simulink model "grid_2021a"  (R2021a)
settings: Solver=VariableStepAuto  StartTime=0.1  StopTime=40  RelTol=1e-3
values from neighbouring files (symbols this model uses):
  close_time = 40    [params.m]
  J_eol = 2*H_tot*P_nom/w_eol_nom^2    (= 921600)    [wind_params.m]
  M1 = M1_backup    [automation.m]    (also in params.m = Machine)
  M2 = M1    [automation.m]    (also in params.m = Machine)
  omega_tab = v_vent_tab*lambda_opt/R_pal    [wind_params.m]
  open_time = 80    [params.m]
  P_eol = P_ren - P_sol    [automation.m]
  P_sol = Power_per_pannel * round((0.6 * P_ren)/ Power_per_pannel)    [automation.m]    (also in params_solar.m = 1000000)
  Pn_L1 = M1.P0 + M2.P0 + P_ren    [automation.m]    (also in params.m = M1.P0 + M2.P0)
  Pn_L2 = Pn_L1 * 0.01    [automation.m]    (also in params.m = Pn_L1 * 0.2)
  Power_per_pannel = 383    [params_battery.m]    (also in params_solar.m = 180.43249709)
  R_pal = 24    [wind_params.m]
  ref_volt = 4160    [params.m]
  ro_air = 1.22    [wind_params.m]
  S_pal = pi*R_pal*R_pal    (= 1809.55736847)    [wind_params.m]
  Ts = 2e-4    (= 0.0002)    [params_solar.m]
  w_eol_nom = v_pal_nom/R_pal    (= 3.125)    [wind_params.m]
  w_zero = 3.000    (= 3)    [wind_params.m]
undefined symbols (not defined in the file or in its folder): Cp_ref, P_eol_base, P_opt_tab2
libraries: nesl_utility x45, fl_lib x43, ee_lib x27
(part 2 of 2)

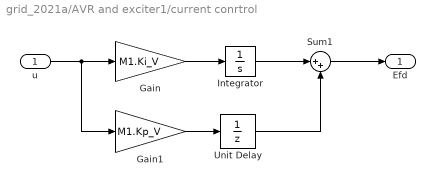
== system grid_2021a/AVR and exciter1/current conrtrol ==
  u : Inport
  Gain : Gain  Gain=M1.Ki_V
  Gain1 : Gain  Gain=M1.Kp_V
  Integrator : Integrator
  Sum1 : Sum  Inputs=|++
  Unit Delay : UnitDelay  InitialCondition=1  SampleTime=-1  HasFrameUpgradeWarning=on
  Efd : Outport
  wires:
  u/1 -> Gain1/1, Gain/1
  Sum1/1 -> Efd/1
  Gain/1 -> Integrator/1
  Integrator/1 -> Sum1/1
  Gain1/1 -> Unit Delay/1
  Unit Delay/1 -> Sum1/2

== system grid_2021a/AVR and exciter2/current conrtrol ==
  u : Inport
  Gain : Gain  Gain=M2.Ki_V
  Gain1 : Gain  Gain=M2.Kp_V
  Integrator : Integrator
  Sum1 : Sum  Inputs=|++
  Unit Delay : UnitDelay  InitialCondition=1  SampleTime=-1  HasFrameUpgradeWarning=on
  Efd : Outport
  wires:
  u/1 -> Gain1/1, Gain/1
  Sum1/1 -> Efd/1
  Gain/1 -> Integrator/1
  Integrator/1 -> Sum1/1
  Gain1/1 -> Unit Delay/1
  Unit Delay/1 -> Sum1/2

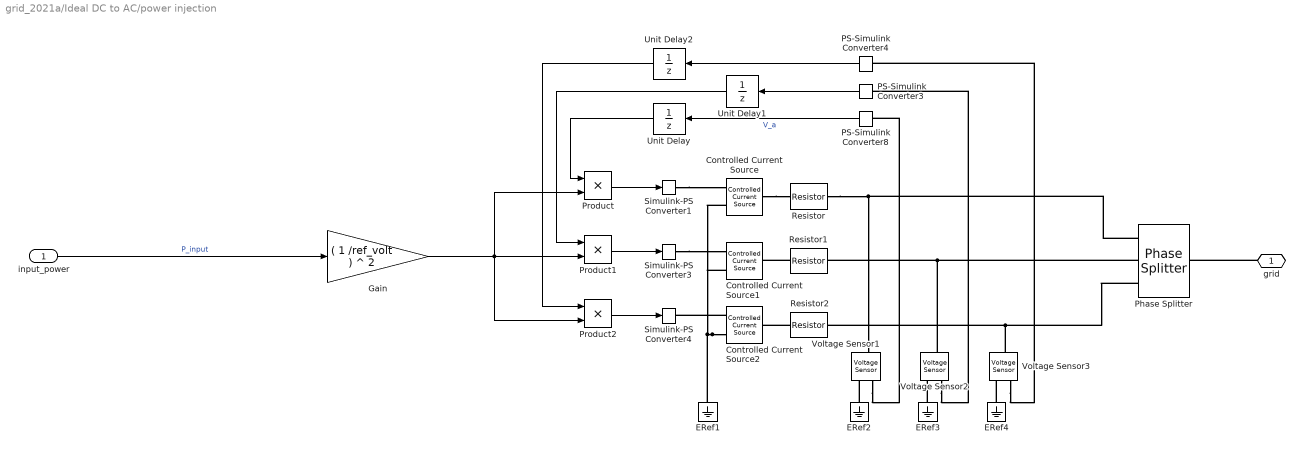
== system grid_2021a/Ideal DC to AC/power injection ==
  input_power : Inport
  Controlled Current Source : fl_lib/Electrical/Electrical Sources/Controlled Current Source
  Controlled Current Source1 : fl_lib/Electrical/Electrical Sources/Controlled Current Source
  Controlled Current Source2 : fl_lib/Electrical/Electrical Sources/Controlled Current Source
  ERef{1..4} (4 alike) : fl_lib/Electrical/Electrical Elements/Electrical Reference
  Gain : Gain  Gain=( 1 /ref_volt ) ^ 2
  PS-Simulink Converter3 : nesl_utility/PS-Simulink Converter  PhysicalDomain=network_engine_domain  SubClassName=ps_output  LeftPortType=input  RightPortType=output  PseudoPeriodic=off  Frequencies=[]  VectorFormat=1-D array  Unit=inherit  AffineConversion=off
  PS-Simulink Converter4 : nesl_utility/PS-Simulink Converter  PhysicalDomain=network_engine_domain  SubClassName=ps_output  LeftPortType=input  RightPortType=output  PseudoPeriodic=off  Frequencies=[]  VectorFormat=1-D array  Unit=inherit  AffineConversion=off
  PS-Simulink Converter8 : nesl_utility/PS-Simulink Converter  PhysicalDomain=network_engine_domain  SubClassName=ps_output  LeftPortType=input  RightPortType=output  PseudoPeriodic=off  Frequencies=[]  VectorFormat=1-D array  Unit=inherit  AffineConversion=off
  Phase Splitter : ee_lib/Connectors & References/Phase Splitter
  Product : Product
  Product1 : Product
  Product2 : Product
  Resistor : fl_lib/Electrical/Electrical Elements/Resistor  R=1e-6 Ohm  i_specify=off  i_priority=None  i=0 A  i_nominal_specify=off  i_nominal_unit=A  i_nominal_value=1  v_specify=off  v_priority=None  v=0 V  v_nominal_specify=off  v_nominal_unit=V  v_nominal_value=1
  Resistor1 : fl_lib/Electrical/Electrical Elements/Resistor  R=1e-6 Ohm  i_specify=off  i_priority=None  i=0 A  i_nominal_specify=off  i_nominal_unit=A  i_nominal_value=1  v_specify=off  v_priority=None  v=0 V  v_nominal_specify=off  v_nominal_unit=V  v_nominal_value=1
  Resistor2 : fl_lib/Electrical/Electrical Elements/Resistor  R=1e-6 Ohm  i_specify=off  i_priority=None  i=0 A  i_nominal_specify=off  i_nominal_unit=A  i_nominal_value=1  v_specify=off  v_priority=None  v=0 V  v_nominal_specify=off  v_nominal_unit=V  v_nominal_value=1
  Simulink-PS Converter1 : nesl_utility/Simulink-PS Converter  PhysicalDomain=network_engine_domain  SubClassName=ps_input  LeftPortType=input  RightPortType=output  PseudoPeriodic=off  Frequencies=[]  NoiseDistribution=none  NoiseParameters=[]  Unit=1  AffineConversion=off  FilteringAndDerivatives=filter  SimscapeFilterOrder=1  InputFilterTimeConstant=0.0001  UdotUserProvided=0
  Simulink-PS Converter3 : nesl_utility/Simulink-PS Converter  PhysicalDomain=network_engine_domain  SubClassName=ps_input  LeftPortType=input  RightPortType=output  PseudoPeriodic=off  Frequencies=[]  NoiseDistribution=none  NoiseParameters=[]  Unit=1  AffineConversion=off  FilteringAndDerivatives=filter  SimscapeFilterOrder=1  InputFilterTimeConstant=0.0001  UdotUserProvided=0
  Simulink-PS Converter4 : nesl_utility/Simulink-PS Converter  PhysicalDomain=network_engine_domain  SubClassName=ps_input  LeftPortType=input  RightPortType=output  PseudoPeriodic=off  Frequencies=[]  NoiseDistribution=none  NoiseParameters=[]  Unit=1  AffineConversion=off  FilteringAndDerivatives=filter  SimscapeFilterOrder=1  InputFilterTimeConstant=0.0001  UdotUserProvided=0
  Unit Delay : UnitDelay  SampleTime=-1  HasFrameUpgradeWarning=on
  Unit Delay1 : UnitDelay  SampleTime=-1  HasFrameUpgradeWarning=on
  Unit Delay2 : UnitDelay  SampleTime=-1  HasFrameUpgradeWarning=on
  Voltage Sensor1 : fl_lib/Electrical/Electrical Sensors/Voltage Sensor
  Voltage Sensor2 : fl_lib/Electrical/Electrical Sensors/Voltage Sensor
  Voltage Sensor3 : fl_lib/Electrical/Electrical Sensors/Voltage Sensor
  grid : PMIOPort  Side=Right
  wires:
  PS-Simulink Converter4/1 -> Unit Delay2/1
  PS-Simulink Converter8/1 -> Unit Delay/1  "V_a"
  PS-Simulink Converter3/1 -> Unit Delay1/1
  Product/1 -> Simulink-PS Converter1/1
  Product1/1 -> Simulink-PS Converter3/1
  Product2/1 -> Simulink-PS Converter4/1
  Unit Delay/1 -> Product/1
  Unit Delay1/1 -> Product1/1
  Unit Delay2/1 -> Product2/1
  Gain/1 -> Product1/2, Product2/2, Product/2
  input_power/1 -> Gain/1  "P_input"
  connections:
  Resistor1/LConn1 -- Controlled Current Source1/LConn1
  Resistor2/LConn1 -- Controlled Current Source2/LConn1
  ERef2/LConn1 -- Voltage Sensor1/RConn2
  Controlled Current Source2/RConn2 -- ERef1/LConn1 -- Controlled Current Source/RConn2 -- Controlled Current Source1/RConn2
  Phase Splitter/RConn1 -- Resistor/RConn1 -- Voltage Sensor1/LConn1
  Simulink-PS Converter1/RConn1 -- Controlled Current Source/RConn1
  ERef4/LConn1 -- Voltage Sensor3/RConn2
  Controlled Current Source/LConn1 -- Resistor/LConn1
  Phase Splitter/RConn2 -- Resistor1/RConn1 -- Voltage Sensor2/LConn1
  Controlled Current Source2/RConn1 -- Simulink-PS Converter4/RConn1
  grid/RConn1 -- Phase Splitter/LConn1
  ERef3/LConn1 -- Voltage Sensor2/RConn2
  Phase Splitter/RConn3 -- Resistor2/RConn1 -- Voltage Sensor3/LConn1
  Simulink-PS Converter3/RConn1 -- Controlled Current Source1/RConn1
  Voltage Sensor1/RConn1 -- PS-Simulink Converter8/LConn1
  Voltage Sensor2/RConn1 -- PS-Simulink Converter3/LConn1
  Voltage Sensor3/RConn1 -- PS-Simulink Converter4/LConn1

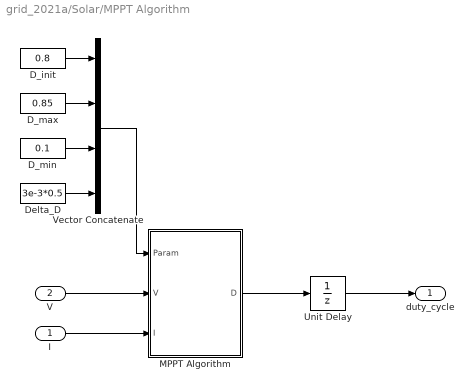
== system grid_2021a/Solar/MPPT Algorithm ==
  I : Inport
  V : Inport  Port=2
  D_init : Constant  Value=0.8
  D_max : Constant  Value=0.85
  D_min : Constant  Value=0.1
  Delta_D : Constant  Value=3e-3*0.5
  MPPT Algorithm : MATLAB Function  SystemSampleTime=Ts
  Unit Delay : UnitDelay  InitialCondition=0.85  SampleTime=-1  HasFrameUpgradeWarning=on
  Vector Concatenate : Concatenate  NumInputs=4
  duty_cycle : Outport
  wires:
  V/1 -> MPPT Algorithm/2(V)
  Vector Concatenate/1 -> MPPT Algorithm/1(Param)
  D_max/1 -> Vector Concatenate/2
  D_init/1 -> Vector Concatenate/1
  D_min/1 -> Vector Concatenate/3
  MPPT Algorithm/1(D) -> Unit Delay/1
  Delta_D/1 -> Vector Concatenate/4
  I/1 -> MPPT Algorithm/3(I)
  Unit Delay/1 -> duty_cycle/1

== system grid_2021a/Solar/Sensing Current ==
  Current Sensor : fl_lib/Electrical/Electrical Sensors/Current Sensor
  PS-Simulink/I : nesl_utility/PS-Simulink Converter  PhysicalDomain=network_engine_domain  SubClassName=ps_output  LeftPortType=input  RightPortType=output  PseudoPeriodic=off  Frequencies=[]  VectorFormat=1-D array  Unit=1  AffineConversion=off
  + : PMIOPort  Side=Left
  - : PMIOPort  Port=2  Side=Right
  I : Outport
  wires:
  PS-Simulink/I/1 -> I/1
  connections:
  -/RConn1 -- Current Sensor/RConn2
  Current Sensor/LConn1 -- +/RConn1
  Current Sensor/RConn1 -- PS-Simulink/I/LConn1

== system grid_2021a/Solar/sensing voltage ==
  PS-Simulink Converter : nesl_utility/PS-Simulink Converter  PhysicalDomain=network_engine_domain  SubClassName=ps_output  LeftPortType=input  RightPortType=output  PseudoPeriodic=off  Frequencies=[]  VectorFormat=1-D array  Unit=inherit  AffineConversion=off
  Voltage Sensor : fl_lib/Electrical/Electrical Sensors/Voltage Sensor
  + : PMIOPort  Side=Left
  - : PMIOPort  Port=2  Side=Right
  V : Outport
  wires:
  PS-Simulink Converter/1 -> V/1
  connections:
  Voltage Sensor/LConn1 -- +/RConn1
  Voltage Sensor/RConn2 -- -/RConn1
  Voltage Sensor/RConn1 -- PS-Simulink Converter/LConn1

== system grid_2021a/Wind turbine/Pitch control ==
  In1 : Inport
  In2 : Inport  Port=2
  Gain1 : Gain  Gain=-200
  Saturation : Saturate  UpperLimit=inf  LowerLimit=0
  Sum1 : Sum  Inputs=|+-
  Out1 : Outport
  wires:
  In2/1 -> Sum1/2
  Gain1/1 -> Saturation/1
  Sum1/1 -> Gain1/1
  In1/1 -> Sum1/1
  Saturation/1 -> Out1/1

== matlab function grid_2021a/Solar/MPPT Algorithm/MPPT Algorithm ==
  settings: updateMethod=DISCRETE  sampleTime=Ts_DC
  data: Param input; V input; I input; D output
function D  = PandO(Param, V, I)

% MPPT controller based on the Perturb & Observe algorithm.

% D output = Duty cycle of the boost converter (value between 0 and 1)
%
% V input = PV array terminal voltage (V)
% I input = PV array current (A)
%
% Param input:
Dinit = Param(1);  %Initial value for D output
Dmax = Param(2);   %Maximum value for D
Dmin = Param(3);   %Minimum value for D
deltaD = Param(4); %Increment value used to increase/decrease the duty cycle D
% ( increasing D = decreasing Vref )
%  

persistent Vold Pold Dold;

if isempty(Vold)
    Vold=0;
    Pold=0;
    Dold=Dinit;
end
P= V*I;
dV= V - Vold;
dP= P - Pold;

if dP ~= 0
    %     if dP>1e-9  & dP<-1e-9 & Enabled ~=0
    if dP < 0
        if dV < 0
            D = Dold - deltaD;
        else
            D = Dold + deltaD;
        end
    else
        if dV < 0
            D = Dold + deltaD;
        else
            D = Dold - deltaD;
        end
    end
else
    D = Dold;
end

if D >= Dmax || D<= Dmin
    D = Dold;
end

Dold = D;
Vold = V;
Pold = P;
